simulink model "complementary_filter"  (R2022b)
settings: Solver=FixedStepAuto  StartTime=0.0  StopTime=90  RelTol=1e-3
values from neighbouring files (symbols this model uses):
  gamma = 0.1    [ModelForCrazyfile.m]    (also in complementary_filter.m = 0.99; myfile.m)
  h = 0.01    [ModelForCrazyfile.m]    (also in complementary_filter.m; linearization.m; myfile.m)
settings Model: Creator=liqui  LastModifiedBy=liqui
settings OptimizationCC: UseDivisionForNetSlopeComputation=on

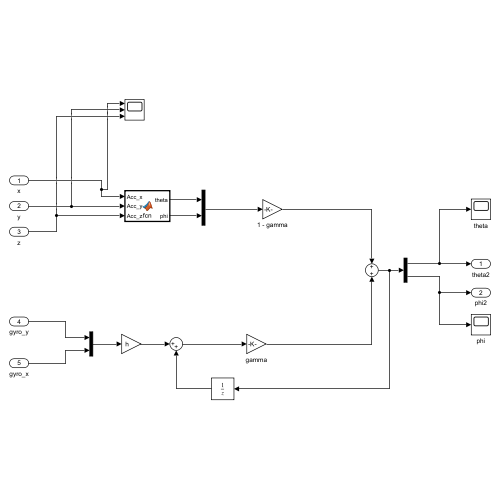
[thumbnail: Simulink's stored preview of the top-level diagram]
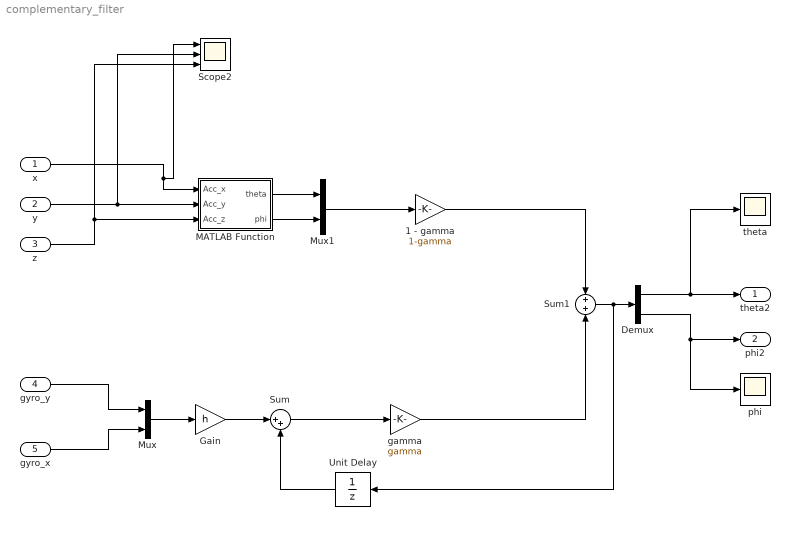
== system complementary_filter ==
  x : Inport
  y : Inport  Port=2
  z : Inport  Port=3
  gyro_y : Inport  Port=4
  gyro_x : Inport  Port=5
  1 - gamma : Gain  Gain=1-gamma
  Demux : Demux  Outputs=2
  Gain : Gain  Gain=h
  MATLAB Function : MATLAB Function  TreatAsAtomicUnit=on
  Mux : Mux  Inputs=2
  Mux1 : Mux  Inputs=2
  Scope2 : Scope  NumInputPorts=3
  Sum : Sum  Inputs=|++
  Sum1 : Sum  Inputs=+|+
  Unit Delay : UnitDelay  SampleTime=-1  HasFrameUpgradeWarning=on
  gamma : Gain  Gain=gamma
  phi : Scope
  theta : Scope
  theta2 : Outport
  phi2 : Outport  Port=2
  wires:
  x/1 -> Scope2/1, MATLAB Function/1(Acc_x)
  z/1 -> MATLAB Function/3(Acc_z), Scope2/3
  y/1 -> MATLAB Function/2(Acc_y), Scope2/2
  Gain/1 -> Sum/1
  Sum/1 -> gamma/1
  gamma/1 -> Sum1/2
  1 - gamma/1 -> Sum1/1
  Unit Delay/1 -> Sum/2
  Mux/1 -> Gain/1
  gyro_x/1 -> Mux/2
  gyro_y/1 -> Mux/1
  MATLAB Function/1(theta) -> Mux1/1
  MATLAB Function/2(phi) -> Mux1/2
  Mux1/1 -> 1 - gamma/1
  Demux/2 -> phi2/1, phi/1
  Demux/1 -> theta2/1, theta/1
  Sum1/1 -> Unit Delay/1, Demux/1

== matlab function complementary_filter/MATLAB Function ==
  data: Acc_x input; theta output; Acc_y input; Acc_z input; phi output
function [theta,phi] = fcn(Acc_x,Acc_y,Acc_z)

theta=atan2(-Acc_x,sqrt(Acc_y.^2+Acc_z.^2));
phi = atan2(Acc_y,Acc_z);

end
